simulink model "bci"  (R2024a)
settings: Solver=VariableStepAuto  StartTime=0.0  StopTime=10.0  RelTol=1e-3
values from neighbouring files (symbols this model uses):
  const_a = Mdl_a.Coeffs(1,2).Const    [RunTime.m]
  ERaw = data{1,1}.X'    [RunTime.m]
  fs = 250    [SaveData.m]    (also in setup.m)
  ind_sel_a = Ia    [OfflineDataAnalysis_Unicorn.m]    (also in RunTime.m = Ia(1:best_feat_a))
  linear_coeffs_a = Mdl_a.Coeffs(1,2).Linear    [RunTime.m]
  shiftLen = 0.20*fs    [RunTime.m]
  winLen = 2*fs    [RunTime.m]
undefined symbols (not defined in the file or in its folder): UN, W1a, W2a
libraries: dspfdesign x34, dspstat3 x2, simulink x2, dspnetwork x1, UnicornLib x1
settings Model: Creator=IRISc  LastModifiedBy=IRISc

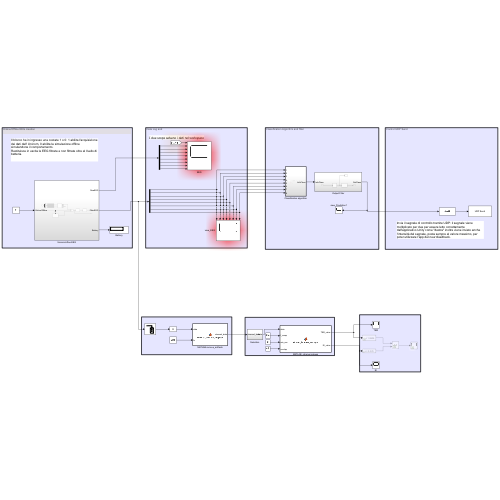
[thumbnail: Simulink's stored preview of the top-level diagram]
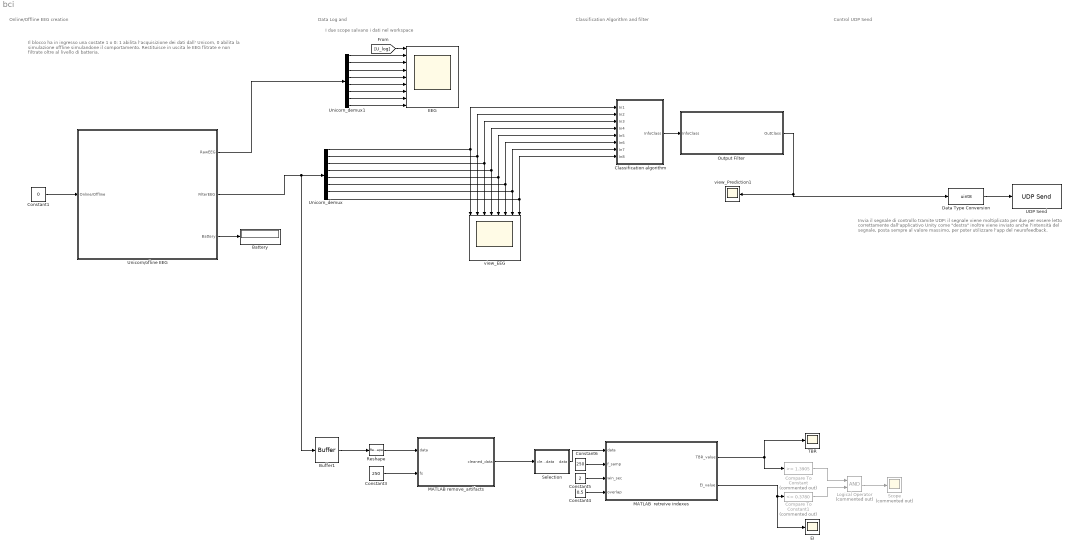
== system bci ==
  note: Invia il segnale di controllo tramite UDP: il segnale viene moltiplicato per due per essere letto correttamente dall'applicativo Unity come "destra" inoltre viene inviato anche l'intensità del segnale, posta sempre al valore massimo, per poter utilizzare l'app del neurofeedback.
  note: Data Log and
  note: Il blocco ha in ingresso una costate 1 o 0: 1 abilita l'acquisizione dei dati dall' Unicorn, 0 abilita la simulazione offline simulandone il comportamento.
      | Restituisce in uscita le EEG flitrate e non filtrate oltre al livello di batteria.
  note: Control UDP Send
  note: I due scope salvano i dati nel workspace
  note: Online/Offline EEG creation
  note: Classification Algorithm and filter
  Battery : Display
  Buffer1 : Buffer  N=2500  OutputFrames=off
  Classification algorithm : Subsystem  TreatAsAtomicUnit=on
  Compare To Constant : simulink/Logic and Bit Operations/Compare To Constant  Commented=on  relop=>=  const=1.3905  OutDataTypeStr=boolean
  Compare To Constant1 : simulink/Logic and Bit Operations/Compare To Constant  Commented=on  relop=<=  const=0.3780  OutDataTypeStr=boolean
  Constant1 : Constant  Value=0
  Constant3 : Constant  Value=250
  Constant4 : Constant  Value=0.5
  Constant5 : Constant  Value=2
  Constant6 : Constant  Value=250
  Data Type Conversion : DataTypeConversion  OutDataTypeStr=uint8  SaturateOnIntegerOverflow=off  RndMeth=Floor
  EEG : Scope  NumInputPorts=9
  EI : Scope
  Logical Operator : Logic  Commented=on  AllPortsSameDT=off  OutDataTypeStr=boolean
  MATLAB  retreive indexes : MATLAB Function  TreatAsAtomicUnit=on
  MATLAB remove_artifacts : MATLAB Function  TreatAsAtomicUnit=on
  Output Filter : Subsystem
  Reshape : Reshape  OutputDimensionality=Customize  OutputDimensions=[2500,8]
  Scope : Scope  Commented=on
  Selection : Subsystem
  TBR : Scope
  UDP Send : dspnetwork/UDP Send  remoteURL='127.0.0.1'  remotePort=5010  localURL='0.0.0.0'  localPortSource=Automatically determine  localPort=-1  sendBufferSize=8192  sampletime=-1  blockPlatform=[]  separateLengthPort=0
  Unicorn/ofline EEG : Subsystem
  Unicorn_demux : Demux  Outputs=8
  Unicorn_demux1 : Demux  Outputs=8
  view_EEG : Scope  NumInputPorts=8
  view_Prediction1 : Scope
  wires:
  Unicorn_demux/3 -> Classification algorithm/3(In3), view_EEG/3
  Unicorn_demux1/1 -> EEG/2
  Unicorn_demux1/4 -> EEG/5
  Unicorn_demux1/2 -> EEG/3
  Unicorn_demux1/7 -> EEG/8
  Unicorn_demux1/5 -> EEG/6
  Unicorn_demux/7 -> Classification algorithm/7(In7), view_EEG/7
  Unicorn_demux1/6 -> EEG/7
  Unicorn_demux1/3 -> EEG/4
  Constant1/1 -> Unicorn/ofline EEG/1(Online/Offline)
  [U_log] -> EEG/1
  Unicorn/ofline EEG/1(RawEEG) -> Unicorn_demux1/1
  Data Type Conversion/1 -> UDP Send/1
  Unicorn_demux1/8 -> EEG/9
  Output Filter/1(OutClass) -> Data Type Conversion/1, view_Prediction1/1
  Unicorn/ofline EEG/3(Battery) -> Battery/1
  Classification algorithm/1(InfoClass) -> Output Filter/1(InfoClass)
  Unicorn_demux/2 -> Classification algorithm/2(In2), view_EEG/2
  Unicorn_demux/1 -> Classification algorithm/1(In1), view_EEG/1
  Unicorn_demux/4 -> Classification algorithm/4(In4), view_EEG/4
  Unicorn_demux/5 -> Classification algorithm/5(In5), view_EEG/5
  Unicorn_demux/8 -> Classification algorithm/8(In8), view_EEG/8
  Unicorn_demux/6 -> Classification algorithm/6(In6), view_EEG/6
  Unicorn/ofline EEG/2(FilterEEG) -> Buffer1/1, Unicorn_demux/1
  Constant6/1 -> MATLAB  retreive indexes/2(f_samp)
  MATLAB  retreive indexes/2(EI_value) -> EI/1, Compare To Constant1/1
  Logical Operator/1 -> Scope/1
  MATLAB remove_artifacts/1(cleaned_data) -> Selection/1(cleaned_data)
  Constant4/1 -> MATLAB  retreive indexes/4(overlap)
  Compare To Constant1/1 -> Logical Operator/2
  Constant3/1 -> MATLAB remove_artifacts/2(fs)
  Selection/1(data) -> MATLAB  retreive indexes/1(data)
  Compare To Constant/1 -> Logical Operator/1
  Constant5/1 -> MATLAB  retreive indexes/3(win_sec)
  MATLAB  retreive indexes/1(TBR_value) -> Compare To Constant/1, TBR/1
  Reshape/1 -> MATLAB remove_artifacts/1(data)
  Buffer1/1 -> Reshape/1

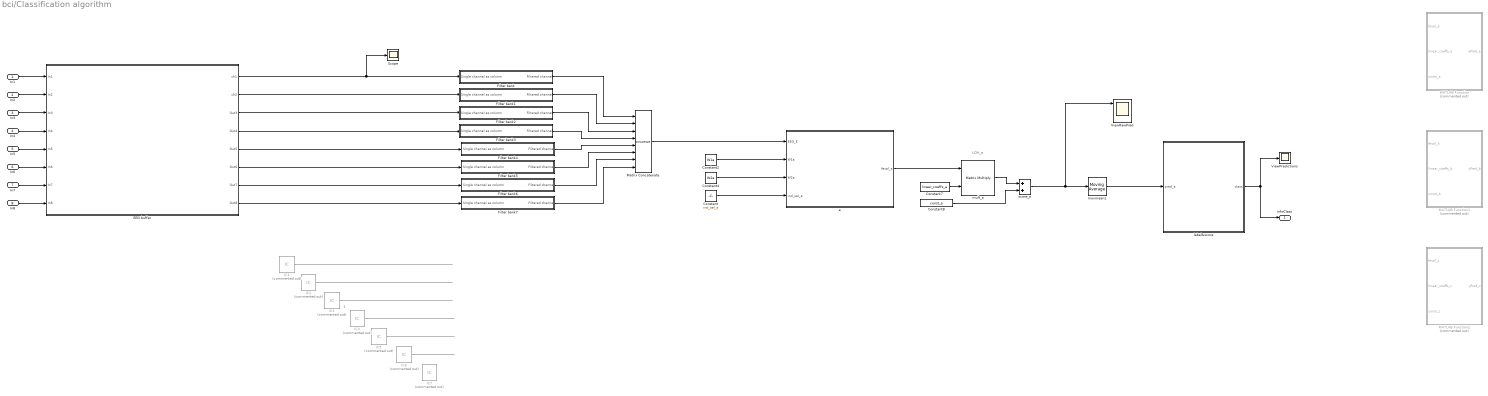
== system bci/Classification algorithm ==
  note: LDA_a
  note: 1
  In1 : Inport
  In2 : Inport  Port=2
  In3 : Inport  Port=3
  In4 : Inport  Port=4
  In5 : Inport  Port=5
  In6 : Inport  Port=6
  In7 : Inport  Port=7
  In8 : Inport  Port=8
  Constant : Constant  Value=ind_sel_a
  Constant2 : Constant  Value=W1a
  Constant4 : Constant  Value=W2a
  Constant7 : Constant  Value=linear_coeffs_a
  Constant8 : Constant  Value=const_a
  EEG buffer : Subsystem
  Filter bank : Subsystem
  Filter bank1 : Subsystem
  Filter bank2 : Subsystem
  Filter bank3 : Subsystem
  Filter bank4 : Subsystem
  Filter bank5 : Subsystem
  Filter bank6 : Subsystem
  Filter bank7 : Subsystem
  IC{1..7} (7 alike) : InitialCondition  Commented=on  Value=0.1
  MATLAB Function : MATLAB Function  Commented=on  TreatAsAtomicUnit=on
  MATLAB Function1 : MATLAB Function  Commented=on  TreatAsAtomicUnit=on
  MATLAB Function2 : MATLAB Function  Commented=on  TreatAsAtomicUnit=on
  Matrix Concatenate : Concatenate  NumInputs=8  Mode=Multidimensional array  ConcatenateDimension=3
  Scope : Scope
  ViewPredictions : Scope
  ViewRawPred : Scope  NumInputPorts=3
  a : MATLAB Function  TreatAsAtomicUnit=on
  label&score : MATLAB Function  TreatAsAtomicUnit=on
  movmean1 : dspstat3/Moving Average  Method=Sliding window  ForgettingFactorPort=off  SpecifyWindowLength=on  WindowLength=3  OverlapLength=2  AllowArbitraryInputLength=off  ForgettingFactor=0.9  SimulateUsing=Code generation
  mult_a : Product  Multiplication=Matrix(*)
  score_a : Sum
  InfoClass : Outport
  wires:
  In1/1 -> EEG buffer/1(In1)
  In2/1 -> EEG buffer/2(In2)
  In3/1 -> EEG buffer/3(In3)
  In4/1 -> EEG buffer/4(In4)
  In5/1 -> EEG buffer/5(In5)
  In6/1 -> EEG buffer/6(In6)
  In7/1 -> EEG buffer/7(In7)
  In8/1 -> EEG buffer/8(In8)
  EEG buffer/1(ch1) -> Scope/1, Filter bank/1(Single channel as column)
  label&score/1(class) -> ViewPredictions/1, InfoClass/1
  Filter bank5/1(Filtered channel) -> Matrix Concatenate/6
  Filter bank6/1(Filtered channel) -> Matrix Concatenate/7
  a/1(feval_a) -> mult_a/1
  Filter bank4/1(Filtered channel) -> Matrix Concatenate/5
  Filter bank1/1(Filtered channel) -> Matrix Concatenate/2
  Filter bank7/1(Filtered channel) -> Matrix Concatenate/8
  Filter bank2/1(Filtered channel) -> Matrix Concatenate/3
  Filter bank3/1(Filtered channel) -> Matrix Concatenate/4
  Filter bank/1(Filtered channel) -> Matrix Concatenate/1
  Matrix Concatenate/1 -> a/1(EEG_E)
  EEG buffer/8(Out8) -> Filter bank7/1(Single channel as column)
  Constant/1 -> a/4(ind_sel_a)
  Constant4/1 -> a/3(W2a)
  Constant2/1 -> a/2(W1a)
  Constant7/1 -> mult_a/2
  Constant8/1 -> score_a/2
  score_a/1 -> ViewRawPred/1, movmean1/1
  mult_a/1 -> score_a/1
  IC1/1 -> ?
  IC4/1 -> ?
  ? -> IC6/1
  IC2/1 -> ?
  ? -> IC2/1
  IC5/1 -> ?
  ? -> IC5/1
  ? -> IC7/1
  ? -> IC4/1
  IC3/1 -> ?
  ? -> IC1/1
  IC6/1 -> ?
  ? -> IC3/1
  EEG buffer/2(ch2) -> Filter bank1/1(Single channel as column)
  EEG buffer/3(Out3) -> Filter bank2/1(Single channel as column)
  EEG buffer/4(Out4) -> Filter bank3/1(Single channel as column)
  EEG buffer/5(Out5) -> Filter bank4/1(Single channel as column)
  EEG buffer/6(Out6) -> Filter bank5/1(Single channel as column)
  EEG buffer/7(Out7) -> Filter bank6/1(Single channel as column)
  movmean1/1 -> label&score/1(pred_a)

== system bci/Output Filter ==
  InfoClass : Inport
  MATLAB Function1 : MATLAB Function  TreatAsAtomicUnit=on
  Moving Average : dspstat3/Moving Average  Method=Sliding window  ForgettingFactorPort=off  SpecifyWindowLength=on  WindowLength=7  OverlapLength=6  AllowArbitraryInputLength=off  ForgettingFactor=0.9  SimulateUsing=Interpreted execution
  Scope : Scope
  OutClass : Outport
  wires:
  Moving Average/1 -> Scope/1, MATLAB Function1/1(u)
  MATLAB Function1/1(y) -> OutClass/1
  InfoClass/1 -> Moving Average/1

== system bci/Selection ==
  cleaned_data : Inport
  Buffer2 : Buffer  N=2500  OutputFrames=off
  Selector : Selector  InputPortWidth=8  IndexOptions=Index vector (dialog)  Indices=[1 3 5]  OutputSizes=1  RuntimeRangeChecks=on
  Unbuffer2 : Unbuffer
  data : Outport
  wires:
  Unbuffer2/1 -> Selector/1
  Selector/1 -> Buffer2/1
  cleaned_data/1 -> Unbuffer2/1
  Buffer2/1 -> data/1

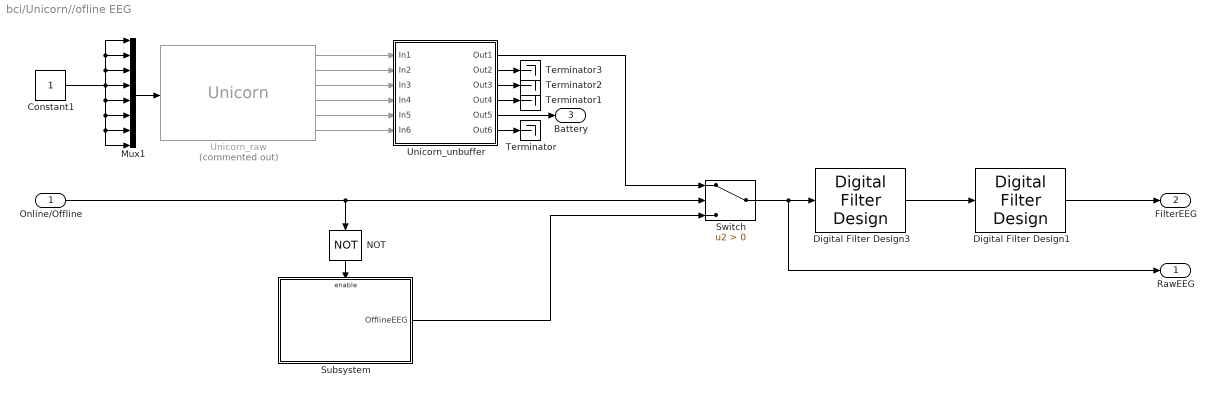
== system bci/Unicorn//ofline EEG ==
  Online/Offline : Inport
  Constant1 : Constant  OutDataTypeStr=boolean
  Digital Filter Design1 : dspfdesign/Digital Filter Design  mwdsp_browser_bugfix_var=off
  Digital Filter Design3 : dspfdesign/Digital Filter Design  mwdsp_browser_bugfix_var=off
  Mux1 : Mux  Inputs=8
  NOT : Logic  Operator=NOT  IconShape=distinctive  AllPortsSameDT=off  OutDataTypeStr=boolean
  Subsystem : Subsystem
  Switch : Switch  Criteria=u2 > Threshold  SaturateOnIntegerOverflow=off  InputSameDT=off
  Terminator{,1..3} (4 alike) : Terminator
  Unicorn_raw : UnicornLib/Unicorn  Commented=on  serial=UN-2023.04.40  old_serial=UN-2023.04.40  frame_length=1  input_source=Electrode
      settings: SourceProductName=Unicorn
  Unicorn_unbuffer : Subsystem
      mask Display:
      | port_label('input',1,'EEG')
      | port_label('input',2,'ACC')
      | port_label('input',3,'GYRO')
      | port_label('input',4,'VALID')
      | port_label('input',5,'BAT')
      | port_label('input',6,'CNT')
      | port_label('output',1,'EEG')
      | port_label('output',2,'ACC')
      | port_label('output',3,'GYRO')
      | port_label('output',4,'VALID')
      | port_label('output',5,'BAT')
      | port_label('output',6,'CNT')
  RawEEG : Outport
  FilterEEG : Outport  Port=2
  Battery : Outport  Port=3
  wires:
  Subsystem/1(OfflineEEG) -> Switch/3
  Mux1/1 -> Unicorn_raw/1
  Unicorn_raw/1 -> Unicorn_unbuffer/1(In1)
  Unicorn_raw/3 -> Unicorn_unbuffer/3(In3)
  Unicorn_raw/5 -> Unicorn_unbuffer/5(In5)
  Digital Filter Design1/1 -> FilterEEG/1
  Unicorn_unbuffer/2(Out2) -> Terminator3/1
  Constant1/1 -> Mux1/2, Mux1/1, Mux1/3, Mux1/5, Mux1/6, Mux1/7, Mux1/8, Mux1/4
  Unicorn_raw/2 -> Unicorn_unbuffer/2(In2)
  Unicorn_raw/4 -> Unicorn_unbuffer/4(In4)
  Unicorn_unbuffer/4(Out4) -> Terminator1/1
  Unicorn_unbuffer/6(Out6) -> Terminator/1
  Digital Filter Design3/1 -> Digital Filter Design1/1
  Unicorn_unbuffer/3(Out3) -> Terminator2/1
  Unicorn_raw/6 -> Unicorn_unbuffer/6(In6)
  Online/Offline/1 -> NOT/1, Switch/2
  Unicorn_unbuffer/1(Out1) -> Switch/1
  Switch/1 -> RawEEG/1, Digital Filter Design3/1
  Unicorn_unbuffer/5(Out5) -> Battery/1
  NOT/1 -> Subsystem/Enable

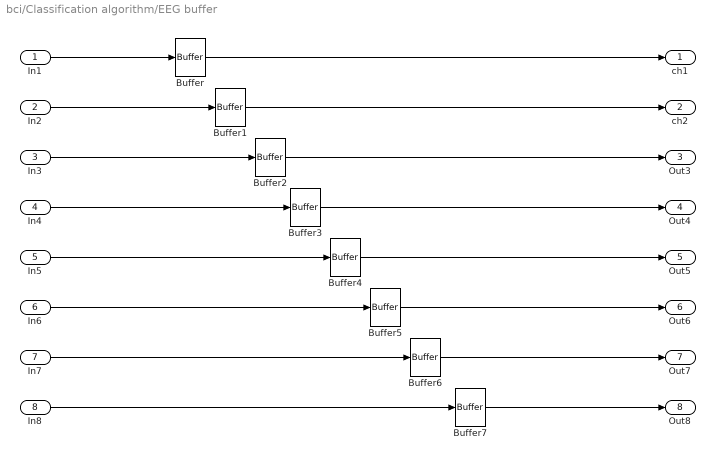
== system bci/Classification algorithm/EEG buffer ==
  In1 : Inport
  In2 : Inport  Port=2
  In3 : Inport  Port=3
  In4 : Inport  Port=4
  In5 : Inport  Port=5
  In6 : Inport  Port=6
  In7 : Inport  Port=7
  In8 : Inport  Port=8
  Buffer{,1..7} (8 alike) : Buffer  N=winLen  V=winLen-floor(shiftLen)  OutputFrames=off
  ch1 : Outport
  ch2 : Outport  Port=2
  Out3 : Outport  Port=3
  Out4 : Outport  Port=4
  Out5 : Outport  Port=5
  Out6 : Outport  Port=6
  Out7 : Outport  Port=7
  Out8 : Outport  Port=8
  wires:
  Buffer/1 -> ch1/1
  In4/1 -> Buffer3/1
  In3/1 -> Buffer2/1
  In5/1 -> Buffer4/1
  Buffer5/1 -> Out6/1
  In1/1 -> Buffer/1
  In2/1 -> Buffer1/1
  Buffer7/1 -> Out8/1
  In7/1 -> Buffer6/1
  Buffer2/1 -> Out3/1
  In8/1 -> Buffer7/1
  Buffer4/1 -> Out5/1
  In6/1 -> Buffer5/1
  Buffer1/1 -> ch2/1
  Buffer3/1 -> Out4/1
  Buffer6/1 -> Out7/1

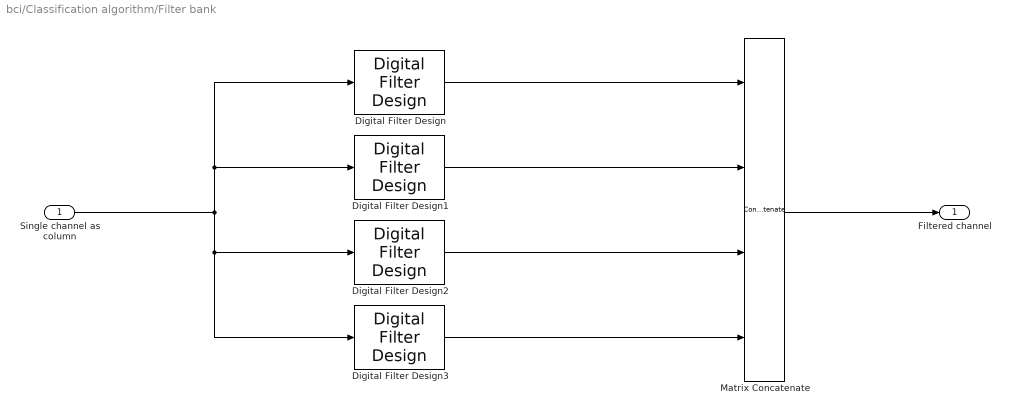
== system bci/Classification algorithm/Filter bank ==
  Single channel as column : Inport
  Digital Filter Design{,1..3} (4 alike) : dspfdesign/Digital Filter Design  mwdsp_browser_bugfix_var=off
  Matrix Concatenate : Concatenate  NumInputs=4  Mode=Multidimensional array  ConcatenateDimension=2
  Filtered channel : Outport  VectorParamsAs1DForOutWhenUnconnected=off
  wires:
  Digital Filter Design1/1 -> Matrix Concatenate/2
  Digital Filter Design3/1 -> Matrix Concatenate/4
  Single channel as column/1 -> Digital Filter Design1/1, Digital Filter Design/1, Digital Filter Design3/1, Digital Filter Design2/1
  Digital Filter Design/1 -> Matrix Concatenate/1
  Digital Filter Design2/1 -> Matrix Concatenate/3
  Matrix Concatenate/1 -> Filtered channel/1

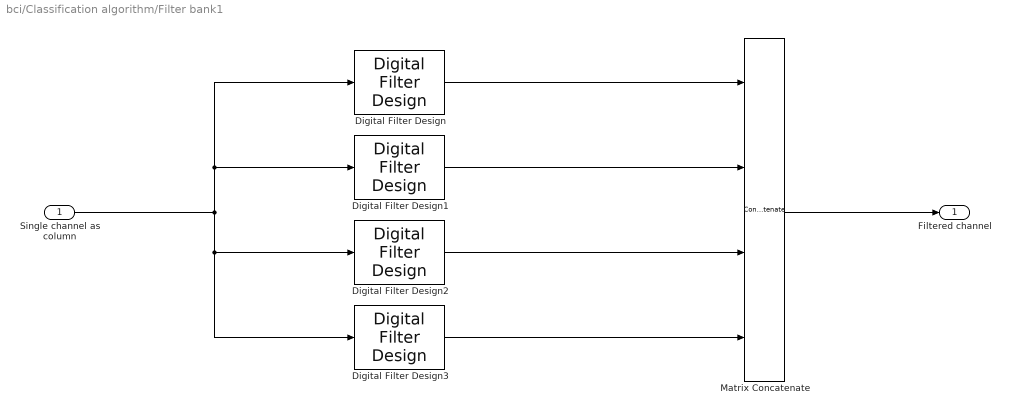
== system bci/Classification algorithm/Filter bank1 ==
  Single channel as column : Inport
  Digital Filter Design{,1..3} (4 alike) : dspfdesign/Digital Filter Design  mwdsp_browser_bugfix_var=off
  Matrix Concatenate : Concatenate  NumInputs=4  Mode=Multidimensional array  ConcatenateDimension=2
  Filtered channel : Outport  VectorParamsAs1DForOutWhenUnconnected=off
  wires:
  Digital Filter Design1/1 -> Matrix Concatenate/2
  Digital Filter Design3/1 -> Matrix Concatenate/4
  Single channel as column/1 -> Digital Filter Design/1, Digital Filter Design1/1, Digital Filter Design2/1, Digital Filter Design3/1
  Digital Filter Design/1 -> Matrix Concatenate/1
  Digital Filter Design2/1 -> Matrix Concatenate/3
  Matrix Concatenate/1 -> Filtered channel/1

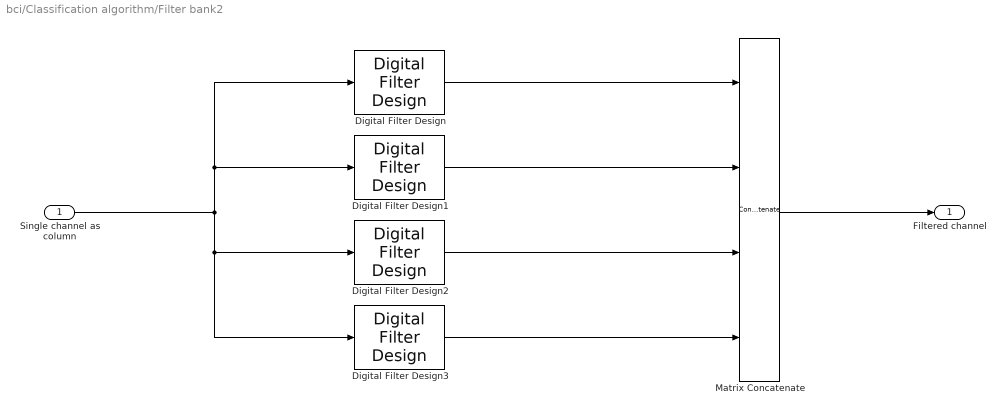
== system bci/Classification algorithm/Filter bank2 ==
  Single channel as column : Inport
  Digital Filter Design{,1..3} (4 alike) : dspfdesign/Digital Filter Design  mwdsp_browser_bugfix_var=off
  Matrix Concatenate : Concatenate  NumInputs=4  Mode=Multidimensional array  ConcatenateDimension=2
  Filtered channel : Outport  VectorParamsAs1DForOutWhenUnconnected=off
  wires:
  Matrix Concatenate/1 -> Filtered channel/1
  Single channel as column/1 -> Digital Filter Design1/1, Digital Filter Design/1, Digital Filter Design3/1, Digital Filter Design2/1
  Digital Filter Design/1 -> Matrix Concatenate/1
  Digital Filter Design3/1 -> Matrix Concatenate/4
  Digital Filter Design2/1 -> Matrix Concatenate/3
  Digital Filter Design1/1 -> Matrix Concatenate/2

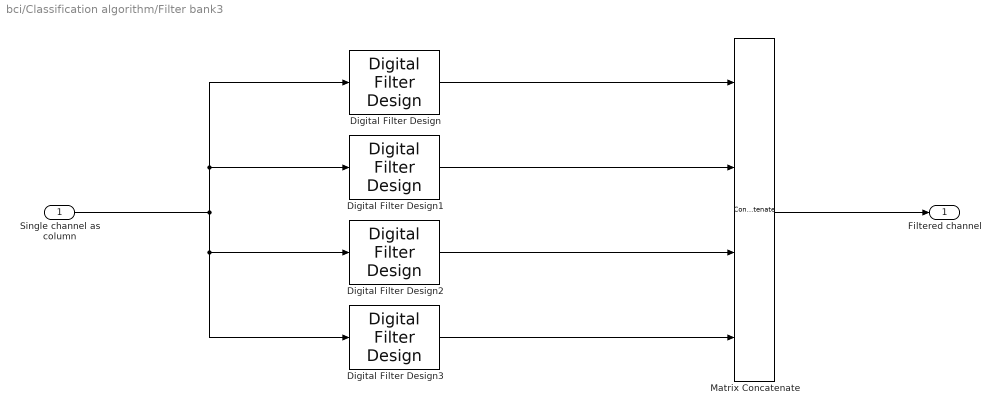
== system bci/Classification algorithm/Filter bank3 ==
  Single channel as column : Inport
  Digital Filter Design{,1..3} (4 alike) : dspfdesign/Digital Filter Design  mwdsp_browser_bugfix_var=off
  Matrix Concatenate : Concatenate  NumInputs=4  Mode=Multidimensional array  ConcatenateDimension=2
  Filtered channel : Outport  VectorParamsAs1DForOutWhenUnconnected=off
  wires:
  Matrix Concatenate/1 -> Filtered channel/1
  Single channel as column/1 -> Digital Filter Design1/1, Digital Filter Design/1, Digital Filter Design2/1, Digital Filter Design3/1
  Digital Filter Design/1 -> Matrix Concatenate/1
  Digital Filter Design3/1 -> Matrix Concatenate/4
  Digital Filter Design2/1 -> Matrix Concatenate/3
  Digital Filter Design1/1 -> Matrix Concatenate/2

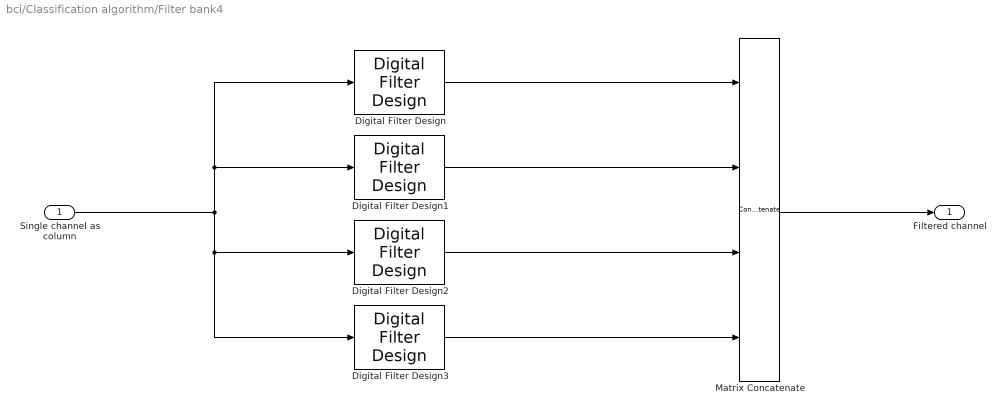
== system bci/Classification algorithm/Filter bank4 ==
  Single channel as column : Inport
  Digital Filter Design{,1..3} (4 alike) : dspfdesign/Digital Filter Design  mwdsp_browser_bugfix_var=off
  Matrix Concatenate : Concatenate  NumInputs=4  Mode=Multidimensional array  ConcatenateDimension=2
  Filtered channel : Outport  VectorParamsAs1DForOutWhenUnconnected=off
  wires:
  Matrix Concatenate/1 -> Filtered channel/1
  Single channel as column/1 -> Digital Filter Design/1, Digital Filter Design1/1, Digital Filter Design2/1, Digital Filter Design3/1
  Digital Filter Design/1 -> Matrix Concatenate/1
  Digital Filter Design3/1 -> Matrix Concatenate/4
  Digital Filter Design2/1 -> Matrix Concatenate/3
  Digital Filter Design1/1 -> Matrix Concatenate/2

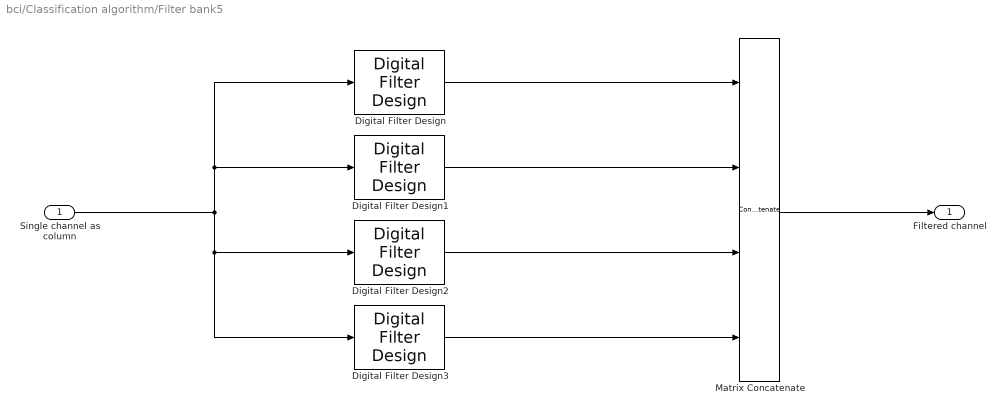
== system bci/Classification algorithm/Filter bank5 ==
  Single channel as column : Inport
  Digital Filter Design{,1..3} (4 alike) : dspfdesign/Digital Filter Design  mwdsp_browser_bugfix_var=off
  Matrix Concatenate : Concatenate  NumInputs=4  Mode=Multidimensional array  ConcatenateDimension=2
  Filtered channel : Outport  VectorParamsAs1DForOutWhenUnconnected=off
  wires:
  Matrix Concatenate/1 -> Filtered channel/1
  Single channel as column/1 -> Digital Filter Design1/1, Digital Filter Design/1, Digital Filter Design2/1, Digital Filter Design3/1
  Digital Filter Design/1 -> Matrix Concatenate/1
  Digital Filter Design3/1 -> Matrix Concatenate/4
  Digital Filter Design2/1 -> Matrix Concatenate/3
  Digital Filter Design1/1 -> Matrix Concatenate/2

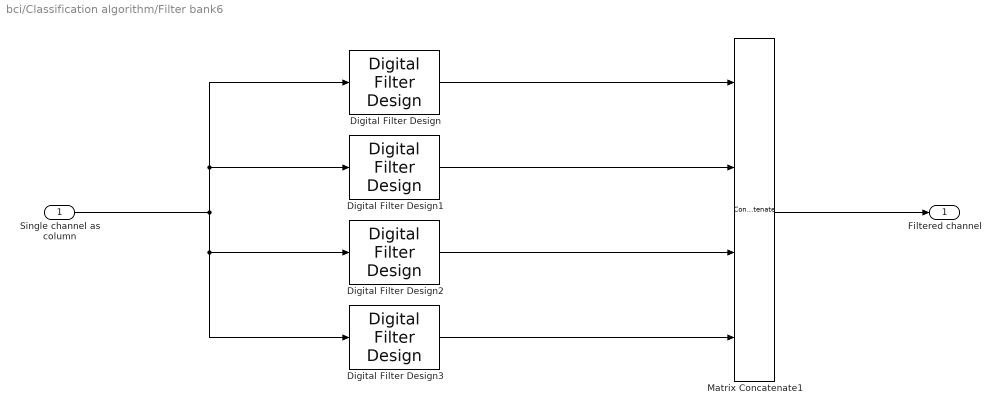
== system bci/Classification algorithm/Filter bank6 ==
  Single channel as column : Inport
  Digital Filter Design{,1..3} (4 alike) : dspfdesign/Digital Filter Design  mwdsp_browser_bugfix_var=off
  Matrix Concatenate1 : Concatenate  NumInputs=4  Mode=Multidimensional array  ConcatenateDimension=2
  Filtered channel : Outport  VectorParamsAs1DForOutWhenUnconnected=off
  wires:
  Matrix Concatenate1/1 -> Filtered channel/1
  Single channel as column/1 -> Digital Filter Design1/1, Digital Filter Design/1, Digital Filter Design3/1, Digital Filter Design2/1
  Digital Filter Design/1 -> Matrix Concatenate1/1
  Digital Filter Design3/1 -> Matrix Concatenate1/4
  Digital Filter Design2/1 -> Matrix Concatenate1/3
  Digital Filter Design1/1 -> Matrix Concatenate1/2

== system bci/Classification algorithm/Filter bank7 ==
  Single channel as column : Inport
  Digital Filter Design{,1..3} (4 alike) : dspfdesign/Digital Filter Design  mwdsp_browser_bugfix_var=off
  Matrix Concatenate : Concatenate  NumInputs=4  Mode=Multidimensional array  ConcatenateDimension=2
  Filtered channel : Outport  VectorParamsAs1DForOutWhenUnconnected=off
  wires:
  Matrix Concatenate/1 -> Filtered channel/1
  Single channel as column/1 -> Digital Filter Design1/1, Digital Filter Design/1, Digital Filter Design3/1, Digital Filter Design2/1
  Digital Filter Design/1 -> Matrix Concatenate/1
  Digital Filter Design3/1 -> Matrix Concatenate/4
  Digital Filter Design2/1 -> Matrix Concatenate/3
  Digital Filter Design1/1 -> Matrix Concatenate/2

== system bci/Unicorn//ofline EEG/Subsystem ==
  Online/Offline : EnablePort
  test_RawEEG1 : Constant  Value=ERaw  SampleTime=(1/fs)*length(ERaw)
  tranpose_test1 : Math  Operator=transpose
  unbuffer_test1 : Unbuffer
  OfflineEEG : Outport
  wires:
  test_RawEEG1/1 -> tranpose_test1/1
  tranpose_test1/1 -> unbuffer_test1/1
  unbuffer_test1/1 -> OfflineEEG/1

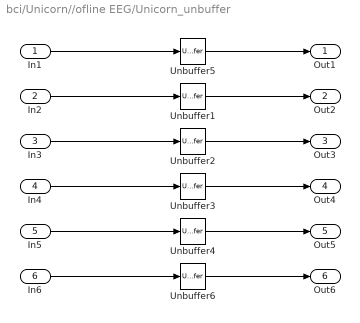
== system bci/Unicorn//ofline EEG/Unicorn_unbuffer ==
  In1 : Inport
  In2 : Inport  Port=2
  In3 : Inport  Port=3
  In4 : Inport  Port=4
  In5 : Inport  Port=5
  In6 : Inport  Port=6
  Unbuffer{1..6} (6 alike) : Unbuffer
  Out1 : Outport
  Out2 : Outport  Port=2
  Out3 : Outport  Port=3
  Out4 : Outport  Port=4
  Out5 : Outport  Port=5
  Out6 : Outport  Port=6
  wires:
  In2/1 -> Unbuffer1/1
  In3/1 -> Unbuffer2/1
  In4/1 -> Unbuffer3/1
  In5/1 -> Unbuffer4/1
  Unbuffer4/1 -> Out5/1
  Unbuffer3/1 -> Out4/1
  Unbuffer2/1 -> Out3/1
  Unbuffer1/1 -> Out2/1
  Unbuffer6/1 -> Out6/1
  In6/1 -> Unbuffer6/1
  In1/1 -> Unbuffer5/1
  Unbuffer5/1 -> Out1/1

== matlab function bci/Classification algorithm/label&score ==
  data: pred_a input; class output
function class = get_class(pred_a)
    % Se il punteggio è positivo o zero, Movimento
    if pred_a >= 0 
        class = 1; 
    % Se il punteggio è negativo, Riposo
    else
        class = 0; 
    end
end

%codice di prima faceva se pred_a>0 e pred_b>0 allora sicuro era sinistra
% classificatore A dice che sei a destra della sua linea E il classificatore B
% dice che sei a destra della sua linea... allora incrociando i dati sei sicuramente la classe Sinistra

% function class = get_class(pred_a, pred_b, pred_c)
%     if ((pred_a>=0) && (pred_b>=0)) %1 left
%         class = -1;
%     elseif ((pred_a<0) && (pred_c>=0)) %2 right
%         class= 1;
%     else %rest
%         class = 0;
%     end
% end


% function class = get_class(pred_a, pred_b, pred_c)
% 
% if ((pred_a==1) && (pred_b==1)) %1 left
%     class = -1;
% elseif ((pred_a==2) && (pred_c==2)) %2 right
%     class= 1;
% else %rest
%     class = 0;
% end
% 
% 
% end

== matlab function bci/Classification algorithm/a ==
  data: EEG_E input; feval_a output; W1a input; W2a input; ind_sel_a input
function feval_a = CSPeval_a(EEG_E,W1a,W2a,ind_sel_a)

EEG_E = permute(EEG_E,[3,1,2]); %dim [8 x 500 x 4]

% CSP

V1a_eval  = CSPapply(EEG_E,[],W1a,W2a,[],[]);

feval_a = V1a_eval(:,ind_sel_a);
% else
%     V1a_eval = zeros(1,24)
% 
%     feval_a = V1a_eval(:,ind_sel_a)
% end


end

== matlab function bci/Classification algorithm/MATLAB Function ==
  data: feval_a input; linear_coeffs_a input; yPred_a output; const_a input
% Calcola i punteggi discriminanti per ogni classe.
function yPred_a = ldaPredict_a(feval_a, linear_coeffs_a, const_a)
    % 'feval_a' è un vettore delle feature in ingresso
    % 'linear_coeffs_a' è una matrice dei coefficienti lineari
    % 'const_a' è un vettore dei bias (intercette)

    score = dot(feval_a, linear_coeffs_a) + const_a; 
    %score = linear_coeffs_a * feval_a + const_a;

    % Predizione: scegli la classe con il punteggio più alto
    if score > 0 
        yPred_a = 1;
    else
        yPred_a = 2;
    end
    
    %prova a dare in uscita lo score e poi lo confronti in get class come
    %fa MicSom
end

== matlab function bci/Output Filter/MATLAB Function1 ==
  data: u input; y output
function y = fcn(u)
persistent u_back ;
u_back = 0 ;
if u >= u_back && u > 0.6
    u_back = u ;
    y = 1 ;
elseif u <= u_back && u < 0.6
    u_back = u ;
    y = 0 ;
elseif u > u_back
    u_back = u ;
    y = 0 ;
else
    u_back = u ;
    y = 1 ;
end

== matlab function bci/MATLAB  retreive indexes ==
  data: data input; TBR_value output; f_samp input; win_sec input; overlap input; EI_value output
function [TBR_value, EI_value] = retrieve_indexes_wrapper(data,f_samp,win_sec, overlap)
    coder.extrinsic('utils.retrieve_indexes_fly');
    TBR_value = double(0);
    EI_value = double(0);
    [TBR_value, EI_value] = utils.retrieve_indexes_fly(data, f_samp, win_sec, overlap);

== matlab function bci/Classification algorithm/MATLAB Function1 ==
  data: feval_b input; linear_coeffs_b input; yPred_b output; const_b input
% Calcola i punteggi discriminanti per ogni classe.
function yPred_b = ldaPredict_b(feval_b, linear_coeffs_b, const_b)
    % 'feval_a' è un vettore delle feature in ingresso
    % 'linear_coeffs_a' è una matrice dei coefficienti lineari
    % 'const_a' è un vettore dei bias (intercette)

    score = dot(feval_b, linear_coeffs_b) + const_b; 
    %score = linear_coeffs_b * feval_b + const_b;

    % Predizione: scegli la classe con il punteggio più alto
    if score > 0 
        yPred_b = 1;
    else
        yPred_b = 3;
    end
    
end

== matlab function bci/Classification algorithm/MATLAB Function2 ==
  data: feval_c input; linear_coeffs_c input; yPred_c output; const_c input
% Calcola i punteggi discriminanti per ogni classe.
function yPred_c  = ldaPredict_c(feval_c, linear_coeffs_c, const_c)
    % 'feval_a' è un vettore delle feature in ingresso
    % 'linear_coeffs_a' è una matrice dei coefficienti lineari
    % 'const_a' è un vettore dei bias (intercette)

    score = dot(feval_c, linear_coeffs_c) + const_c; 
    %score = linear_coeffs_c * feval_c + const_c;

    % Predizione: scegli la classe con il punteggio più alto
    if score > 0 
        yPred_c = 2;
    else
        yPred_c = 3;
    end
    
end

== matlab function bci/MATLAB remove_artifacts ==
  data: data input; cleaned_data output; fs input
function cleaned_data = remove_artifacts_wrapper(data, fs)
    coder.extrinsic('utils.remove_artifacts_eeg_fly');

    cleaned_data = zeros(2500, 8); 
    cleaned_data = utils.remove_artifacts_eeg_fly(data, fs);
end
